simulink model "IEEE_1547_UI_TEST"  (R2018b)
settings: Solver=ode4  StartTime=0.0  StopTime=inf  FixedStep=Ts  RelTol=1e-3  EnableMultiTasking=on
PostLoadFcn:
  | Ts=40e-6; ARTEMIS_DISABLE_RTLAB_COMPATIBILTY_CHECK=1;
InitFcn:
  | Ts=40e-6; ARTEMIS_DISABLE_RTLAB_COMPATIBILTY_CHECK=1;
undefined symbols (not defined in the file or in its folder): another_event_name, I, Left, my_event_name, Right, type, V
libraries: simulink x72, powerlib_meascontrol x70, powerlib x66, artemis x4, rtlab x3, rtio_opalrt_ml605ex1 x3
(part 1 of 3)
Description:
  | Model of a simple control system for use iin training.
settings Model: ARTEMISmethode_block_infos=$$__separator__$$IEEE_P1547_TEST_V22/ARTEMIS Guide$$__separator__$$  Creator=Paul Baracos  LastModifiedBy=DETLDAQ
settings DataIOCC: LimitDataPoints=on  SaveFormat=Array  SaveOutput=off  SaveTime=off  SignalLoggingName=sigsOut
settings OptimizationCC: BlockReduction=off  BooleanDataType=off  OptimizeBlockIOStorage=off  BufferReuse=off  GlobalBufferReuse=off  ExpressionFolding=off  LocalBlockOutputs=off  InitFltsAndDblsToZero=on  LifeSpan=inf  OptimizeDataStoreBuffers=off  BusAssignmentInplaceUpdate=off
settings DebuggingCC: SaveWithParameterizedLinksMsg=none  UnderspecifiedInitializationDetection=Classic  MergeDetectMultiDrivingBlocksExec=none  SignalResolutionControl=TryResolveAllWithWarning  MultiTaskDSMMsg=warning  MultiTaskCondExecSysMsg=none  FcnCallInpInsideContextMsg=warning  SFUnexpectedBacktrackingDiag=warning  SFNoUnconditionalDefaultTransitionDiag=warning  SFExecutionAtInitializationDiag=none
settings HardwareCC: ProdBitPerPointer=32  ProdBitPerSizeT=32  ProdBitPerPtrDiffT=32  ProdLargestAtomicFloat=None  ProdIntDivRoundTo=Undefined  ProdEndianess=Unspecified  ProdWordSize=32  ProdHWDeviceType=32-bit Generic  TargetBitPerPointer=64  TargetBitPerSizeT=64  TargetBitPerPtrDiffT=64  TargetLongLongMode=on  TargetIntDivRoundTo=Zero  TargetEndianess=LittleEndian  TargetWordSize=64  TargetHWDeviceType=MATLAB Host  ProdEqTarget=off
settings ModelReferenceCC: PropagateSignalLabelsOutOfModel=off
settings SFSimCC: SimUseLocalCustomCode=off
settings RTWCC: Description=Generic Real-Time Target  RTWUseLocalCustomCode=off
settings CodeAppCC: StateflowObjectComments=on
settings GRTTargetCC: TargetFcnLib=ansi_tfl_tmw.mat  TargetLangStandard=C89/C90 (ANSI)  GeneratePreprocessorConditionals=Disable all  CombineOutputUpdateFcns=off  GRTInterface=on
settings ConfigComp: CovMetricSettings=dw  CovHtmlReporting=on  CovSaveCumulativeToWorkspaceVar=on  CovSaveSingleToWorkspaceVar=on  CovExternalEMLEnable=off

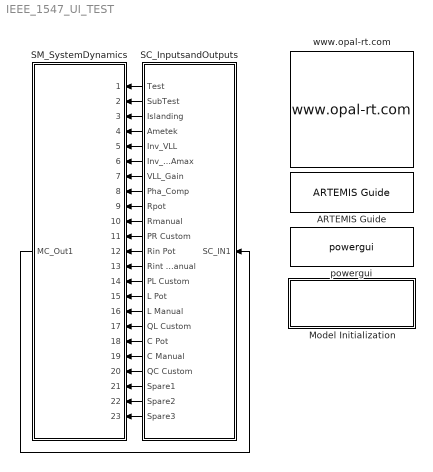
== system IEEE_1547_UI_TEST ==
  ARTEMIS Guide : artemis/ARTEMIS/ARTEMIS Guide  Tag=FTSSmethode_opal_4hx0r99  Description=5.0_z1  lock=on  Ts=Ts  ssn=on  opt=art5  dyna=off  nb_perm=4  RT_fullcomp=off  ssn_itvc=off  ssn_ivic=off  ssn_ext=off  ssn_solver=Backward Euler  iter_type=iSWITCH and iMOV only (default)  ssn_ImpulseLoopBlockedStateUpdate=5  ssn_mov_iter_number=5  ssn_switch_iter_number=5  ssn_lu_or_ldlt=LU (more robust)  ssn_nib_type_verify=on  ssn_use_lu=on  ssn_use_ldlt=off  ssn_impulse=on  ssn_quasimpulse=off  ssn_impulse_loop=5  paraExtinctionThy=off  Thy_Impulse=off  dtc=Off  dtc_opt=normal  ao=on  simtype=off  ct_mac=off  lin_mov=off  lsp=[0.001 2]  spike_skip=Disabled  dtc_extra=1  dtc_sws=normal  dtc_pied=0.5  SPSRulesBlock=SPSRules  tre=off  ctmm=off  LF=on  dpl_type=ARTEMiS DPL  rlc_type=off  custom_type=off  para=on  ssn_full_iteration=off
  Model Initialization : Subsystem  AncestorBlock=artemis/Tools /Misc/Model Initialization  mask(Model Functions){InitFcnX=Ts=40e-6; ARTEMIS_DISABLE_RTLAB_COMPATIBILTY_CHECK=1;, prel=off, posl=on, inif=on, strf=off}
      mask prompts: InitFcnX "Initialisation"; prel "Preload Function"; posl "PostLoad Function"; inif "InitFcn"; strf "StartFcn"
      mask init:
      | currentBlock = gcb;
      | root = bdroot(currentBlock);
      | 
      | if ~strcmp(get_param(root,'BlockDiagramType'),'library')
      |     if prel==1
      |         set_param(root, 'PreLoadFcn', InitFcnX);
      |     else
      |         set_param(root, 'PreLoadFcn', '');
      |     end
      |     if inif==1
      |         set_param(root, 'InitFcn', InitFcnX);
      |     else
      |         set_param(root, 'InitFcn', '');
      |     end
      |     if strf==1
      |         set_param(root, 'StartFcn', InitFcnX);
      |     else
      |         set_param(root, 'StartFcn', '');
      |     end
      |     if posl==1
      |         set_param(root, 'PostLoadFcn', InitFcnX);
      |     else
      |         set_param(root, 'PostLoadFcn', '');
      |     end
      | end
      | 
      | pos = get_param(currentBlock, 'Position');
      | width = pos(3) - pos(1); height = pos(4) - pos(2);
      | txt = [ upper(root) '\n' '- InitFcn. . . . . '  get_param(root, 'InitFcn') ];
      settings: CopyFcn=set_param(gcb,'LinkStatus','inactive')
      mask Display: text(5, height*0.5, txt, 'horizontalAlignment', 'left', 'verticalAlignment', 'middle') ;
  SC_InputsandOutputs : Subsystem
  SM_SystemDynamics : Subsystem
  powergui : powerlib/powergui  Priority=1  SimulationMode=Discrete  SampleTime=Ts  frequency=60  Iterations=50  frequencyindice=60  Pbase=100e6  ErrMax=1e-4  UnitsV=kV  UnitsW=MW  buscounter=0  FunctionMessages=off  echomessages=off  EnableUseOfTLC=off  CurrentSourceSwitches=off  DisableSnubberDevices=off  DisableRonSwitches=off  DisableVfSwitches=off  DisplayEquations=off  SolverType=Tustin/Backward Euler (TBE)  Interpol=off  ExternalGateDelay=off  methode=off  Ts=10  x0status=blocks  SPID=off  SwTol=0  HookPort=off  RestoreLinks=warning  ResistiveCurrentMeasurement=off  Frange=[0:2:500]  Ylog=off  Xlog=on  ShowGrid=off  save=off  variable=ZData  structure=0  ZoomFFT=off  StartTime=0.0  cycles=1  DisplayStyle=1  fundamental=60  FreqAxis=off  MaxFrequency=1000  frequencyindicesteady=1  RmsSteady=1  display=off
  www.opal-rt.com : artemis/Internal/www.opal-rt.com  SystemSampleTime=-1
  wires:
  SM_SystemDynamics/1(MC_Out1) -> SC_InputsandOutputs/1(SC_IN1)
  SC_InputsandOutputs/1(Test) -> SM_SystemDynamics/1(" 1")
  SC_InputsandOutputs/2(SubTest) -> SM_SystemDynamics/2(" 2")
  SC_InputsandOutputs/3(Islanding) -> SM_SystemDynamics/3(" 3")
  SC_InputsandOutputs/4(Ametek) -> SM_SystemDynamics/4(" 4")
  SC_InputsandOutputs/5(Inv_VLL) -> SM_SystemDynamics/5(" 5")
  SC_InputsandOutputs/6(Inv_KVAmax) -> SM_SystemDynamics/6(" 6")
  SC_InputsandOutputs/7(VLL_Gain) -> SM_SystemDynamics/7(" 7")
  SC_InputsandOutputs/8(Pha_Comp) -> SM_SystemDynamics/8(" 8")
  SC_InputsandOutputs/9(Rpot) -> SM_SystemDynamics/9(" 9")
  SC_InputsandOutputs/10(Rmanual) -> SM_SystemDynamics/10(" 10")
  SC_InputsandOutputs/11(PR Custom) -> SM_SystemDynamics/11(" 11")
  SC_InputsandOutputs/12(Rin Pot) -> SM_SystemDynamics/12(" 12")
  SC_InputsandOutputs/13(Rint Manual) -> SM_SystemDynamics/13(" 13")
  SC_InputsandOutputs/14(PL Custom) -> SM_SystemDynamics/14(" 14")
  SC_InputsandOutputs/15(L Pot) -> SM_SystemDynamics/15(" 15")
  SC_InputsandOutputs/16(L Manual) -> SM_SystemDynamics/16(" 16")
  SC_InputsandOutputs/17(QL Custom) -> SM_SystemDynamics/17(" 17")
  SC_InputsandOutputs/18(C Pot) -> SM_SystemDynamics/18(" 18")
  SC_InputsandOutputs/19(C Manual) -> SM_SystemDynamics/19(" 19")
  SC_InputsandOutputs/20(QC Custom) -> SM_SystemDynamics/20(" 20")
  SC_InputsandOutputs/21(Spare1) -> SM_SystemDynamics/21(" 21")
  SC_InputsandOutputs/22(Spare2) -> SM_SystemDynamics/22(" 22")
  SC_InputsandOutputs/23(Spare3) -> SM_SystemDynamics/23(" 23")

== system IEEE_1547_UI_TEST/Model Initialization ==

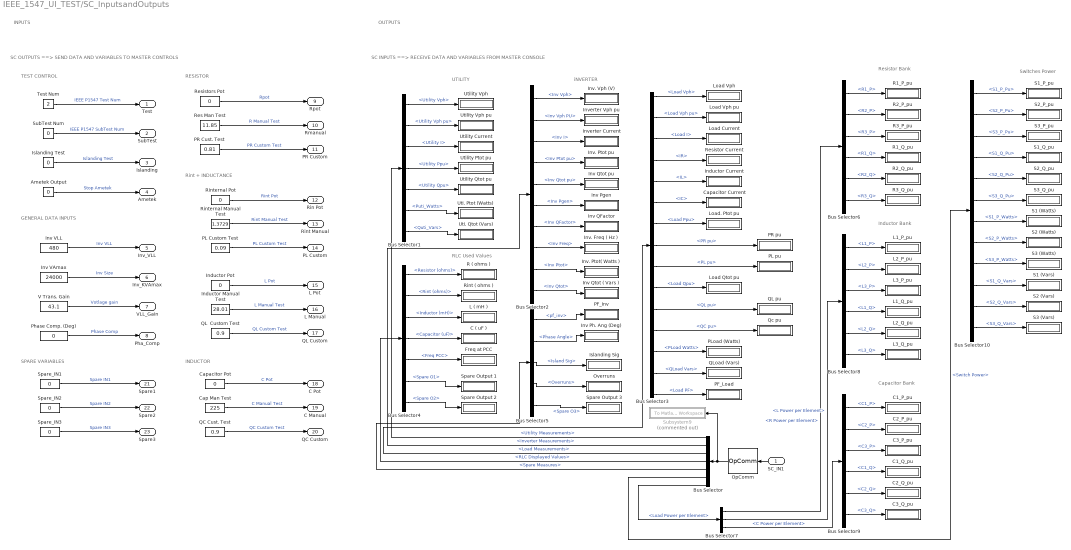
== system IEEE_1547_UI_TEST/SC_InputsandOutputs ==
  note: INPUTS
  note: RLC Used Values
  note: iNVERTER
  note: UTILITY
  note: SC INPUTS ==> RECEIVE DATA AND VARIABLES FROM MASTER CONSOLE
  note: TEST CONTROL
  note: SC OUTPUTS ==> SEND DATA AND VARIABLES TO MASTER CONTROLS
  note: INDUCTOR
  note: RESISTOR
  note: GENERAL DATA INPUTS
  note: Rint + INDUCTANCE
  note: SPARE VARIABLES
  note: OUTPUTS
  note: Resistor Bank
  note: Inductor Bank
  note: Capacitor Bank
  note: Switches Power
  SC_IN1 : Inport
  " PF_Load" : Display
  Ametek Output : Constant  Value=0
  Bus Selector : BusSelector  OutputSignals=Utility Measurements,Inverter Measurements,Load Measurements,RLC Displayed Values,Spare Measures,Switch Power,Load Power per Element
  Bus Selector1 : BusSelector  OutputSignals=Utility Vph,Utility Vph pu,Utility I,Utility Ppu,Utility Qpu,Puti_Watts,Quti_Vars
  Bus Selector10 : BusSelector  OutputSignals=S1_P_Pu,S2_P_Pu,S3_P_Pu,S1_Q_Pu,S2_Q_Pu,S3_Q_Pu,S1_P_Watts,S2_P_Watts,S3_P_Watts,S1_Q_Vars,S2_Q_Vars,S3_Q_Vars
  Bus Selector2 : BusSelector  OutputSignals=Inv Vph,Inv Vph PU,Inv I,Inv Ptot pu,Inv Qtot pu,Inv Pgen,Inv QFactor,Inv Freq,Inv Ptot,Inv Qtot
  Bus Selector3 : BusSelector  OutputSignals=Load Vph,Load Vph pu,Load I,IR,IL,IC,Load Ppu,PR pu,PL pu,Load Qpu,QL pu,QC pu,PLoad Watts,QLoad Vars,Load PF
  Bus Selector4 : BusSelector  OutputSignals=Resistor (ohms),Rint (ohms),Inductor (mH),Capacitor (uF),Freq PCC,Spare O1,Spare O2
  Bus Selector5 : BusSelector  OutputSignals=pf_inv,Phase Angle,Island Sig,Overruns,Spare O3
  Bus Selector6 : BusSelector  OutputSignals=R1_P,R2_P,R3_P,R1_Q,R2_Q,R3_Q
  Bus Selector7 : BusSelector  OutputSignals=R Power per Element,L Power per Element,C Power per Element
  Bus Selector8 : BusSelector  OutputSignals=L1_P,L2_P,L3_P,L1_Q,L2_Q,L3_Q
  Bus Selector9 : BusSelector  OutputSignals=C1_P,C2_P,C3_P,C1_Q,C2_Q,C3_Q
  C ( uF ) : Display
  C1_P_pu : Display
      settings: Format=bank
  C1_Q_pu : Display
  C2_P_pu : Display
  C2_Q_pu : Display
  C3_P_pu : Display
      settings: Format=bank
  C3_Q_pu : Display
      settings: Format=bank
  Cap Man Test : Constant  Value=225
  Capacitor Current : Display
      settings: Format=bank
  Capacitor Pot : Constant  Value=0
  Freq at PCC : Display
      settings: Format=bank
  Inductor Current : Display
      settings: Format=bank
  Inductor Manual Test : Constant  Value=28.01
  Inductor Pot : Constant  Value=0
  Inv Pgen : Display
  Inv Ph. Ang (Deg) : Display
  Inv QFactor : Display
  Inv Qtot ( Vars ) : Display
      settings: Format=bank
  Inv Qtot pu : Display
  Inv VAmax : Constant  Value=24000
  Inv VLL : Constant  Value=480
  Inv. Freq ( Hz ) : Display
      settings: Format=bank
  Inv. Ptot pu : Display
  Inv. Ptot( Watts ) : Display
      settings: Format=bank
  Inv. Vph (V) : Display
      settings: Format=bank
  Inverter Current : Display
      settings: Format=bank
  Inverter Vph pu : Display
  Islanding Sig : Display
  Islanding Test : Constant  Value=0
  L ( mH ) : Display
  L1_P_pu : Display
      settings: Format=bank
  L1_Q_pu : Display
  L2_P_pu : Display
  L2_Q_pu : Display
  L3_P_pu : Display
      settings: Format=bank
  L3_Q_pu : Display
      settings: Format=bank
  Load Current : Display
      settings: Format=bank
  Load Qtot pu : Display
  Load Vph : Display
      settings: Format=bank
  Load Vph pu : Display
  Load. Ptot pu : Display
  OpComm : rtlab/OpComm  nbport=1  groupe_acq=1  subsys_rate=0  st=0  Synchronization=on  Interpolation=on  Threshold=1.0  Missed_Data=off  Sim_Time=off  Samples=off  dynSigOut=off  from_console=0  warning_done=off  writeOpCommFile=off  Offset=off
      settings: SourceProductName=RT-LAB
  Overruns : Display
  PF_Inv : Display
  PL Custom Test : Constant  Value=0.09
  PL pu : Display
  PLoad (Watts) : Display
      settings: Format=bank
  PR Cust. Test : Constant  Value=0.81
  PR pu : Display
  Phase Comp. (Deg) : Constant  Value=0
  QC Cust. Test : Constant  Value=0.9
  QL  Custom Test : Constant  Value=0.9
  QL pu : Display
  QLoad (Vars) : Display
      settings: Format=bank
  Qc pu : Display
  R ( ohms ) : Display
  R1_P_pu : Display
      settings: Format=bank
  R1_Q_pu : Display
  R2_P_pu : Display
  R2_Q_pu : Display
  R3_P_pu : Display
      settings: Format=bank
  R3_Q_pu : Display
      settings: Format=bank
  Res Man Test : Constant  Value=11.85
  Resistor Current : Display
      settings: Format=bank
  Resistors Pot : Constant  Value=0
  Rint ( ohms ) : Display
  Rinternal Manual Test : Constant  Value=1.3729
  Rinternal Pot : Constant  Value=0
  S1 (Vars) : Display
  S1 (Watts) : Display
      settings: Format=bank
  S1_P_pu : Display
      settings: Format=bank
  S1_Q_pu : Display
  S2 (Vars) : Display
  S2 (Watts) : Display
      settings: Format=bank
  S2_P_pu : Display
      settings: Format=bank
  S2_Q_pu : Display
  S3 (Vars) : Display
      settings: Format=bank
  S3 (Watts) : Display
  S3_P_pu : Display
  S3_Q_pu : Display
      settings: Format=bank
  Spare Output 1 : Display
  Spare Output 2 : Display
  Spare Output 3 : Display
  Spare_IN1 : Constant  Value=0
  Spare_IN2 : Constant  Value=0
  Spare_IN3 : Constant  Value=0
  SubTest Num : Constant  Value=0
  Subsystem9 : Subsystem  Commented=on
  Test Num : Constant  Value=2
  Uti. Ptot (Watts) : Display
      settings: Format=bank
  Uti. Qtot (Vars) : Display
      settings: Format=bank
  Utility Current : Display
      settings: Format=bank
  Utility Ptot pu : Display
  Utility Qtot pu : Display
  Utility Vph : Display
      settings: Format=bank
  Utility Vph pu : Display
  V Trans. Gain : Constant  Value=43.1
  Test : Outport
  SubTest : Outport  Port=2
  Islanding : Outport  Port=3
  Ametek : Outport  Port=4
  Inv_VLL : Outport  Port=5
  Inv_KVAmax : Outport  Port=6
  VLL_Gain : Outport  Port=7
  Pha_Comp : Outport  Port=8
  Rpot : Outport  Port=9
  Rmanual : Outport  Port=10
  PR Custom : Outport  Port=11
  Rin Pot : Outport  Port=12
  Rint Manual : Outport  Port=13
  PL Custom : Outport  Port=14
  L Pot : Outport  Port=15
  L Manual : Outport  Port=16
  QL Custom : Outport  Port=17
  C Pot : Outport  Port=18
  C Manual : Outport  Port=19
  QC Custom : Outport  Port=20
  Spare1 : Outport  Port=21
  Spare2 : Outport  Port=22
  Spare3 : Outport  Port=23
  wires:
  SC_IN1/1 -> OpComm/1
  Bus Selector/1 -> Bus Selector1/1  "<Utility Measurements>"
  Bus Selector/2 -> Bus Selector2/1  "<Inverter Measurements>"
  Bus Selector/3 -> Bus Selector3/1  "<Load Measurements>"
  Bus Selector/4 -> Bus Selector4/1  "<RLC Displayed Values>"
  Bus Selector/5 -> Bus Selector5/1  "<Spare Measures>"
  Capacitor Pot/1 -> C Pot/1  "C Pot"
  QL  Custom Test/1 -> QL Custom/1  "QL Custom Test"
  Inductor Pot/1 -> L Pot/1  "L Pot"
  Res Man Test/1 -> Rmanual/1  "R Manual Test"
  PR Cust. Test/1 -> PR Custom/1  "PR Custom Test"
  Inductor Manual Test/1 -> L Manual/1  "L Manual Test"
  Rinternal Pot/1 -> Rin Pot/1  "Rint Pot"
  PL Custom Test/1 -> PL Custom/1  "PL Custom Test"
  Resistors Pot/1 -> Rpot/1  "Rpot"
  Rinternal Manual Test/1 -> Rint Manual/1  "Rint Manual Test"
  QC Cust. Test/1 -> QC Custom/1  "QC Custom Test"
  Cap Man Test/1 -> C Manual/1  "C Manual Test"
  Test Num/1 -> Test/1  "IEEE P1547 Test Num"
  SubTest Num/1 -> SubTest/1  "IEEE P1547 SubTest Num"
  Ametek Output/1 -> Ametek/1  "Stop Ametek"
  Islanding Test/1 -> Islanding/1  "Islanding Test"
  V Trans. Gain/1 -> VLL_Gain/1  "Votlage gain"
  Phase Comp. (Deg)/1 -> Pha_Comp/1  "Phase Comp"
  Inv VLL/1 -> Inv_VLL/1  "Inv VLL"
  Inv VAmax/1 -> Inv_KVAmax/1  "Inv Size"
  Spare_IN3/1 -> Spare3/1  "Spare IN3"
  Spare_IN1/1 -> Spare1/1  "Spare IN1"
  Spare_IN2/1 -> Spare2/1  "Spare IN2"
  Bus Selector1/2 -> Utility Vph pu/1  "<Utility Vph pu>"
  Bus Selector1/7 -> Uti. Qtot (Vars)/1  "<Quti_Vars>"
  Bus Selector1/6 -> Uti. Ptot (Watts)/1  "<Puti_Watts>"
  Bus Selector1/4 -> Utility Ptot pu/1  "<Utility Ppu>"
  Bus Selector1/3 -> Utility Current/1  "<Utility I>"
  Bus Selector1/5 -> Utility Qtot pu/1  "<Utility Qpu>"
  Bus Selector1/1 -> Utility Vph/1  "<Utility Vph>"
  Bus Selector2/6 -> Inv Pgen/1  "<Inv Pgen>"
  Bus Selector2/2 -> Inverter Vph pu/1  "<Inv Vph PU>"
  Bus Selector2/3 -> Inverter Current/1  "<Inv I>"
  Bus Selector2/9 -> Inv. Ptot( Watts )/1  "<Inv Ptot>"
  Bus Selector2/7 -> Inv QFactor/1  "<Inv QFactor>"
  Bus Selector2/10 -> Inv Qtot ( Vars )/1  "<Inv Qtot>"
  Bus Selector2/8 -> Inv. Freq ( Hz )/1  "<Inv Freq>"
  Bus Selector2/1 -> Inv. Vph (V)/1  "<Inv Vph>"
  Bus Selector2/4 -> Inv. Ptot pu/1  "<Inv Ptot pu>"
  Bus Selector2/5 -> Inv Qtot pu/1  "<Inv Qtot pu>"
  Bus Selector3/6 -> Capacitor Current/1  "<IC>"
  Bus Selector3/4 -> Resistor Current/1  "<IR>"
  Bus Selector3/7 -> Load. Ptot pu/1  "<Load Ppu>"
  Bus Selector3/15 -> " PF_Load"/1  "<Load PF>"
  Bus Selector3/10 -> Load Qtot pu/1  "<Load Qpu>"
  Bus Selector3/2 -> Load Vph pu/1  "<Load Vph pu>"
  Bus Selector3/3 -> Load Current/1  "<Load I>"
  Bus Selector3/9 -> PL pu/1  "<PL pu>"
  Bus Selector3/5 -> Inductor Current/1  "<IL>"
  Bus Selector3/11 -> QL pu/1  "<QL pu>"
  Bus Selector3/1 -> Load Vph/1  "<Load Vph>"
  Bus Selector3/12 -> Qc pu/1  "<QC pu>"
  Bus Selector3/8 -> PR pu/1  "<PR pu>"
  Bus Selector4/4 -> C ( uF )/1  "<Capacitor (uF)>"
  Bus Selector4/1 -> R ( ohms )/1  "<Resistor (ohms)>"
  Bus Selector4/3 -> L ( mH )/1  "<Inductor (mH)>"
  Bus Selector4/2 -> Rint ( ohms )/1  "<Rint (ohms)>"
  Bus Selector5/3 -> Islanding Sig/1  "<Island Sig>"
  Bus Selector5/5 -> Spare Output 3/1  "<Spare O3>"
  Bus Selector5/2 -> Inv Ph. Ang (Deg)/1  "<Phase Angle>"
  Bus Selector5/1 -> PF_Inv/1  "<pf_inv>"
  OpComm/1 -> Subsystem9/1(" To Matlab Workspace"), Bus Selector/1
  Bus Selector5/4 -> Overruns/1  "<Overruns>"
  Bus Selector4/5 -> Freq at PCC/1  "<Freq PCC>"
  Bus Selector4/6 -> Spare Output 1/1  "<Spare O1>"
  Bus Selector4/7 -> Spare Output 2/1  "<Spare O2>"
  Bus Selector3/13 -> PLoad (Watts)/1  "<PLoad Watts>"
  Bus Selector3/14 -> QLoad (Vars)/1  "<QLoad Vars>"
  Bus Selector7/1 -> Bus Selector6/1  "<R Power per Element>"
  Bus Selector6/6 -> R3_Q_pu/1  "<R3_Q>"
  Bus Selector8/6 -> L3_Q_pu/1  "<L3_Q>"
  Bus Selector/6 -> Bus Selector10/1  "<Switch Power>"
  Bus Selector6/1 -> R1_P_pu/1  "<R1_P>"
  Bus Selector8/4 -> L1_Q_pu/1  "<L1_Q>"
  Bus Selector7/3 -> Bus Selector9/1  "<C Power per Element>"
  Bus Selector7/2 -> Bus Selector8/1  "<L Power per Element>"
  Bus Selector8/1 -> L1_P_pu/1  "<L1_P>"
  Bus Selector9/4 -> C1_Q_pu/1  "<C1_Q>"
  Bus Selector9/5 -> C2_Q_pu/1  "<C2_Q>"
  Bus Selector9/1 -> C1_P_pu/1  "<C1_P>"
  Bus Selector6/2 -> R2_P_pu/1  "<R2_P>"
  Bus Selector6/3 -> R3_P_pu/1  "<R3_P>"
  Bus Selector6/4 -> R1_Q_pu/1  "<R1_Q>"
  Bus Selector8/5 -> L2_Q_pu/1  "<L2_Q>"
  Bus Selector9/2 -> C2_P_pu/1  "<C2_P>"
  Bus Selector8/3 -> L3_P_pu/1  "<L3_P>"
  Bus Selector8/2 -> L2_P_pu/1  "<L2_P>"
  Bus Selector9/6 -> C3_Q_pu/1  "<C3_Q>"
  Bus Selector9/3 -> C3_P_pu/1  "<C3_P>"
  Bus Selector6/5 -> R2_Q_pu/1  "<R2_Q>"
  Bus Selector/7 -> Bus Selector7/1  "<Load Power per Element>"
  Bus Selector10/5 -> S2_Q_pu/1  "<S2_Q_Pu>"
  Bus Selector10/2 -> S2_P_pu/1  "<S2_P_Pu>"
  Bus Selector10/11 -> S2 (Vars)/1  "<S2_Q_Vars>"
  Bus Selector10/4 -> S1_Q_pu/1  "<S1_Q_Pu>"
  Bus Selector10/8 -> S2 (Watts)/1  "<S2_P_Watts>"
  Bus Selector10/3 -> S3_P_pu/1  "<S3_P_Pu>"
  Bus Selector10/9 -> S3 (Watts)/1  "<S3_P_Watts>"
  Bus Selector10/10 -> S1 (Vars)/1  "<S1_Q_Vars>"
  Bus Selector10/1 -> S1_P_pu/1  "<S1_P_Pu>"
  Bus Selector10/12 -> S3 (Vars)/1  "<S3_Q_Vars>"
  Bus Selector10/6 -> S3_Q_pu/1  "<S3_Q_Pu>"
  Bus Selector10/7 -> S1 (Watts)/1  "<S1_P_Watts>"

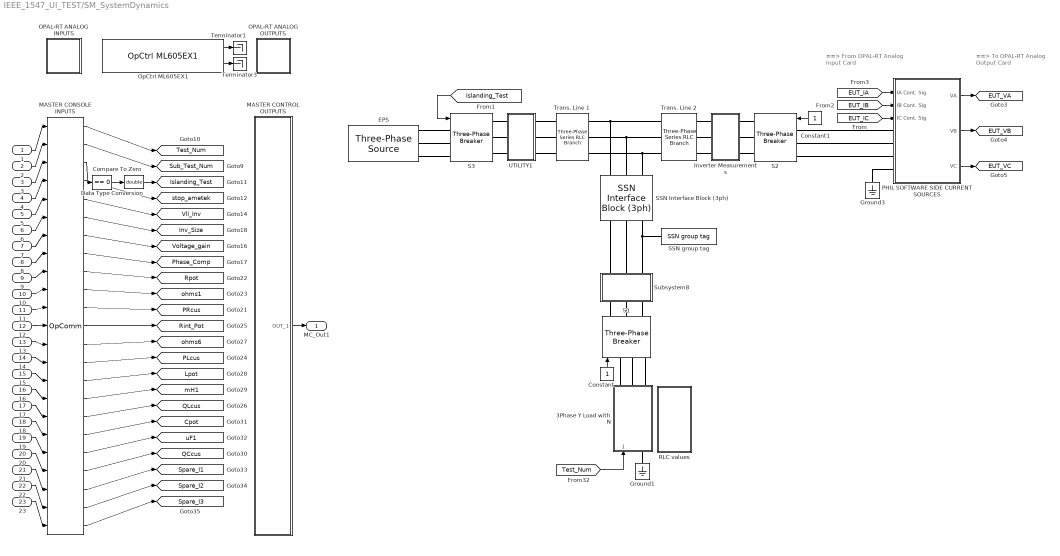
== system IEEE_1547_UI_TEST/SM_SystemDynamics ==
  note: ==> From OPAL-RT
      | Analog Input
      | Card
  note: ==> To OPAL-RT
      | Analog Output
      | Card
  " 1" : Inport
  " 2" : Inport  Port=2
  " 3" : Inport  Port=3
  " 4" : Inport  Port=4
  " 5" : Inport  Port=5
  " 6" : Inport  Port=6
  " 7" : Inport  Port=7
  " 8" : Inport  Port=8
  " 9" : Inport  Port=9
  " 10" : Inport  Port=10
  " 11" : Inport  Port=11
  " 12" : Inport  Port=12
  " 13" : Inport  Port=13
  " 14" : Inport  Port=14
  " 15" : Inport  Port=15
  " 16" : Inport  Port=16
  " 17" : Inport  Port=17
  " 18" : Inport  Port=18
  " 19" : Inport  Port=19
  " 20" : Inport  Port=20
  " 21" : Inport  Port=21
  " 22" : Inport  Port=22
  " 23" : Inport  Port=23
  " 3Phase Y Load with N" : Subsystem
      mask Display:
      | color('blue');
      | disp('3Phase\nY Load\nwith N\n\n');
  " EPS " : powerlib/Electrical Sources/Three-Phase Source  InternalConnection=Yg  VoltagePhases=off  Voltage=480  PhaseAngle=0  Voltage_phases=[613 613 613]/sqrt(3)  PhaseAngles_phases=[30 -90 +150]  Frequency=60  NonIdealSource=on  SpecifyImpedance=on  Resistance=0.002957  Inductance=0.000031  ShortCircuitLevel=1e6  BaseVoltage=480  XRratio=7  BusType=swing  Pref=10e3  Qref=0  Prefabc=[10e3, 10e3, 10e3]  Qrefabc=[0, 0, 0]  Qmin=-inf  Qmax=inf
      settings: SourceProductName=Simscape Electrical
  Compare To Zero : simulink/Logic and Bit Operations/Compare To Zero  relop===  OutDataTypeStr=boolean
  Constant : Constant
  Constant1 : Constant
  Data Type Conversion : DataTypeConversion  OutDataTypeStr=double
  Ground1 : powerlib/Elements/Ground  LConnTagsString=a
      settings: SourceProductName=Simscape Electrical
  Ground3 : powerlib/Elements/Ground  LConnTagsString=a
      settings: SourceProductName=Simscape Electrical
  Inverter Measurements : Subsystem
      mask Display:
      | % color('blue')
      | % disp('Inverter\nMeasurements')
  MASTER CONSOLE INPUTS : rtlab/OpComm  nbport=23  groupe_acq=1  subsys_rate=0  st=0  Synchronization=on  Interpolation=on  Threshold=1.0  Missed_Data=off  Sim_Time=off  Samples=off  dynSigOut=off  from_console=1  warning_done=off  writeOpCommFile=off  Offset=off
      settings: SourceProductName=RT-LAB
  MASTER CONTROL OUTPUTS : Subsystem
  OPAL-RT ANALOG INPUTS : Subsystem
      mask Display:
      | color('red')
      | disp('\nOpal-RT\n\n\n')
      | color('blue')
      | disp('\nAI\nCard')
  OPAL-RT ANALOG OUTPUTS : Subsystem
      mask Display:
      | color('red')
      | disp('\nOpal-RT\n\n\n')
      | color('blue')
      | disp('\nAO\nCard')
  OpCtrl ML605EX1 : rtio_opalrt_ml605ex1/OpCtrl ML605EX1  CtrlName='ML605EX1 Ctrl'  boardid=0  BitstreamFilename=ML605_2-EX-0029-2_3_7_140-32Ao_16Ai_32DioSelectable_C3C1C3FBFBEA-01-05.bin  numconfig=-1  mode=Master  externalClock=off  decimRtsi=0  calibIO=off  SampleTime=0  loadinport=-1
  PHIL SOFTWARE SIDE CURRENT SOURCES : Subsystem
      mask Display:
      | color('blue')
      | disp('\nPHIL\nInverter')
      | color('red')
      | disp('\n\n\n\n\n\nY Grounded\nNeutral')
  RLC values : Subsystem
      mask Display:
      | color('blue')
      | disp('RLC\nValues')
  S1 : powerlib/Elements/Three-Phase Breaker  InitialState=closed  SwitchA=on  SwitchB=on  SwitchC=on  SwitchTimes="[1/60  5/60]"  External=on  BreakerResistance=0.01  SnubberResistance=1e6  SnubberCapacitance=inf  Measurements=None
      settings: SourceProductName=Simscape Electrical
  S2 : powerlib/Elements/Three-Phase Breaker  InitialState=closed  SwitchA=on  SwitchB=on  SwitchC=on  SwitchTimes="[1/60  5/60]"  External=on  BreakerResistance=0.01  SnubberResistance=1e6  SnubberCapacitance=inf  Measurements=None
      settings: SourceProductName=Simscape Electrical
  "S3 " : powerlib/Elements/Three-Phase Breaker  InitialState=closed  SwitchA=on  SwitchB=on  SwitchC=on  SwitchTimes="[1/60  5/60]"  External=on  BreakerResistance=0.01  SnubberResistance=1e6  SnubberCapacitance=inf  Measurements=None
      settings: SourceProductName=Simscape Electrical
  SSN Interface Block (3ph) : artemis/SSN/Nodal Interface Blocks/SSN Interface Block (3ph)  nb_phase=3  nb_port=2  p1_type=V-type(Left)  p2_type=I-type(Right)  p3_type=V-type(Left)  p4_type=V-type(Left)  p5_type=V-type(Left)  p6_type=V-type(Left)  p7_type=V-type(Left)  p8_type=V-type(Left)  p9_type=V-type(Left)  p10_type=V-type(Left)  p11_type=V-type(Left)  p12_type=V-type(Left)  p13_type=V-type(Left)  p14_type=V-type(Left)  p15_type=V-type(Left)  p16_type=V-type(Left)  I_port_shunt_resistance=1e9
  SSN group tag : artemis/SSN/SSN group tag  ssn_group_tag=Group2
  Subsystem8 : Subsystem
  Terminator1 : Terminator
  Terminator3 : Terminator
  Trans. Line 1 : powerlib/Elements/Three-Phase Series RLC Branch  LConnTagsString=A|B|C  RConnTagsString=A|B|C  BranchType=R  Resistance=0.014875  Inductance=0.0000855  Capacitance=1e-6  Measurements=None
      settings: SourceProductName=Simscape Electrical
  Trans. Line 2 : powerlib/Elements/Three-Phase Series RLC Branch  LConnTagsString=A|B|C  RConnTagsString=A|B|C  BranchType=R  Resistance=0.014875  Inductance=0.0000855  Capacitance=0  Measurements=None
      settings: SourceProductName=Simscape Electrical
  UTILITY1 : Subsystem
      mask Display:
      | % color('blue')
      | % disp('Utility\n\n')
      | % color('red')
      | % disp('\nY Grounded\nNeutral')
  MC_Out1 : Outport
  tag scope: Cpot=global, EUT_VA=global, EUT_VB=global, EUT_VC=global, Inv_Size=global, Islanding_Test=global, Lpot=global, PLcus=global, PRcus=global, Phase_Comp=global, QCcus=global, QLcus=global, Rint_Pot=global, Rpot=global, Spare_I1=global, Spare_I2=global, Spare_I3=global, Sub_Test_Num=global, Test_Num=global, Vll_Inv=global, Voltage_gain=global, mH1=global, ohms1=global, ohms6=global, stop_ametek=global, uF1=global
  wires:
  [Islanding_Test] -> "S3 "/1
  OpCtrl ML605EX1/1 -> Terminator1/1
  OpCtrl ML605EX1/2 -> Terminator3/1
  [EUT_IB] -> PHIL SOFTWARE SIDE CURRENT SOURCES/2(IB Cont. Sig)
  PHIL SOFTWARE SIDE CURRENT SOURCES/1(VA) -> [EUT_VA]
  PHIL SOFTWARE SIDE CURRENT SOURCES/2(VB) -> [EUT_VB]
  PHIL SOFTWARE SIDE CURRENT SOURCES/3(VC) -> [EUT_VC]
  [EUT_IA] -> PHIL SOFTWARE SIDE CURRENT SOURCES/1(IA Cont. Sig)
  [EUT_IC] -> PHIL SOFTWARE SIDE CURRENT SOURCES/3(IC Cont. Sig)
  [Test_Num] -> " 3Phase Y Load with N"/1(Test Sel.)
  " 1"/1 -> MASTER CONSOLE INPUTS/1
  " 4"/1 -> MASTER CONSOLE INPUTS/4
  " 2"/1 -> MASTER CONSOLE INPUTS/2
  " 3"/1 -> MASTER CONSOLE INPUTS/3
  " 5"/1 -> MASTER CONSOLE INPUTS/5
  " 6"/1 -> MASTER CONSOLE INPUTS/6
  " 7"/1 -> MASTER CONSOLE INPUTS/7
  " 8"/1 -> MASTER CONSOLE INPUTS/8
  " 9"/1 -> MASTER CONSOLE INPUTS/9
  " 10"/1 -> MASTER CONSOLE INPUTS/10
  " 11"/1 -> MASTER CONSOLE INPUTS/11
  " 12"/1 -> MASTER CONSOLE INPUTS/12
  " 13"/1 -> MASTER CONSOLE INPUTS/13
  " 14"/1 -> MASTER CONSOLE INPUTS/14
  " 15"/1 -> MASTER CONSOLE INPUTS/15
  " 16"/1 -> MASTER CONSOLE INPUTS/16
  " 17"/1 -> MASTER CONSOLE INPUTS/17
  " 18"/1 -> MASTER CONSOLE INPUTS/18
  " 19"/1 -> MASTER CONSOLE INPUTS/19
  " 20"/1 -> MASTER CONSOLE INPUTS/20
  " 21"/1 -> MASTER CONSOLE INPUTS/21
  " 22"/1 -> MASTER CONSOLE INPUTS/22
  " 23"/1 -> MASTER CONSOLE INPUTS/23
  MASTER CONSOLE INPUTS/1 -> [Test_Num]
  MASTER CONSOLE INPUTS/2 -> [Sub_Test_Num]
  MASTER CONSOLE INPUTS/4 -> [stop_ametek]
  MASTER CONSOLE INPUTS/5 -> [Vll_Inv]
  MASTER CONSOLE INPUTS/6 -> [Inv_Size]
  MASTER CONSOLE INPUTS/7 -> [Voltage_gain]
  MASTER CONSOLE INPUTS/8 -> [Phase_Comp]
  MASTER CONSOLE INPUTS/9 -> [Rpot]
  MASTER CONSOLE INPUTS/10 -> [ohms1]
  MASTER CONSOLE INPUTS/11 -> [PRcus]
  MASTER CONSOLE INPUTS/12 -> [Rint_Pot]
  MASTER CONSOLE INPUTS/13 -> [ohms6]
  MASTER CONSOLE INPUTS/14 -> [PLcus]
  MASTER CONSOLE INPUTS/15 -> [Lpot]
  MASTER CONSOLE INPUTS/16 -> [mH1]
  MASTER CONSOLE INPUTS/17 -> [QLcus]
  MASTER CONSOLE INPUTS/18 -> [Cpot]
  MASTER CONSOLE INPUTS/19 -> [uF1]
  MASTER CONSOLE INPUTS/20 -> [QCcus]
  MASTER CONSOLE INPUTS/21 -> [Spare_I1]
  MASTER CONSOLE INPUTS/22 -> [Spare_I2]
  MASTER CONSOLE INPUTS/23 -> [Spare_I3]
  MASTER CONTROL OUTPUTS/1("OUT_1 ") -> MC_Out1/1
  MASTER CONSOLE INPUTS/3 -> Compare To Zero/1
  Compare To Zero/1 -> Data Type Conversion/1
  Data Type Conversion/1 -> [Islanding_Test]
  Constant/1 -> S1/1
  Constant1/1 -> S2/1
  connections:
  Trans. Line 1/RConn1 -- Trans. Line 2/LConn1 -- SSN Interface Block (3ph)/LConn1
  Trans. Line 2/LConn2 -- Trans. Line 1/RConn2 -- SSN Interface Block (3ph)/LConn2
  Trans. Line 2/LConn3 -- Trans. Line 1/RConn3 -- SSN Interface Block (3ph)/LConn3
  Trans. Line 2/RConn1 -- Inverter Measurements/RConn1
  S2/RConn2 -- Inverter Measurements/LConn2
  Trans. Line 2/RConn2 -- Inverter Measurements/RConn2
  S2/RConn3 -- Inverter Measurements/LConn3
  Trans. Line 2/RConn3 -- Inverter Measurements/RConn3
  Ground3/LConn1 -- PHIL SOFTWARE SIDE CURRENT SOURCES/LConn4
  Subsystem8/LConn1 -- SSN Interface Block (3ph)/RConn1
  Subsystem8/LConn2 -- SSN Interface Block (3ph)/RConn2
  SSN group tag/LConn1 -- SSN Interface Block (3ph)/RConn3 -- Subsystem8/LConn3
  Ground1/LConn1 -- " 3Phase Y Load with N"/LConn1
  Subsystem8/RConn1 -- S1/RConn1
  Subsystem8/RConn2 -- S1/RConn2
  Subsystem8/RConn3 -- S1/RConn3
  S2/RConn1 -- Inverter Measurements/LConn1
  " 3Phase Y Load with N"/RConn1 -- S1/LConn1
  " 3Phase Y Load with N"/RConn2 -- S1/LConn2
  " 3Phase Y Load with N"/RConn3 -- S1/LConn3
  "S3 "/LConn1 -- " EPS "/RConn1
  "S3 "/LConn2 -- " EPS "/RConn2
  "S3 "/LConn3 -- " EPS "/RConn3
  UTILITY1/RConn1 -- Trans. Line 1/LConn1
  UTILITY1/RConn2 -- Trans. Line 1/LConn2
  UTILITY1/RConn3 -- Trans. Line 1/LConn3
  UTILITY1/LConn1 -- "S3 "/RConn1
  UTILITY1/LConn2 -- "S3 "/RConn2
  UTILITY1/LConn3 -- "S3 "/RConn3
  S2/LConn1 -- PHIL SOFTWARE SIDE CURRENT SOURCES/LConn1
  S2/LConn2 -- PHIL SOFTWARE SIDE CURRENT SOURCES/LConn2
  S2/LConn3 -- PHIL SOFTWARE SIDE CURRENT SOURCES/LConn3

== system IEEE_1547_UI_TEST/SC_InputsandOutputs/Subsystem9 ==
  " To Matlab Workspace" : Inport
  Bus Selector : BusSelector  OutputSignals=Utility Measurements,Inverter Measurements,Load Measurements,RLC Display Values
  Subsystem5 : Subsystem
  Subsystem6 : Subsystem
  Subsystem7 : Subsystem
  Subsystem8 : Subsystem
  wires:
  " To Matlab Workspace"/1 -> Bus Selector/1
  Bus Selector/2 -> Subsystem6/1(Inverter Measurements)  "<Inverter Measurements>"
  Bus Selector/1 -> Subsystem5/1(Utility Measurements)  "<Utility Measurements>"
  Bus Selector/3 -> Subsystem7/1(Load Measurements)  "<Load Measurements>"
  Bus Selector/4 -> Subsystem8/1(RLC Display Values)  "<RLC Display Values>"

== system IEEE_1547_UI_TEST/SM_SystemDynamics/ 3Phase Y Load with N ==
  Test Sel. : Inport
  "   C Bank" : Subsystem
  "   R Bank1" : Subsystem
  ( Rint + L ) Bank : Subsystem
  3Ph CB Normal : powerlib/Elements/Three-Phase Breaker  InitialState=closed  SwitchA=on  SwitchB=on  SwitchC=on  SwitchTimes="[1/60  5/60]"  External=on  BreakerResistance=0.01  SnubberResistance=1e6  SnubberCapacitance=inf  Measurements=None
      settings: SourceProductName=Simscape Electrical
  3Ph CB Test 1 : powerlib/Elements/Three-Phase Breaker  InitialState=closed  SwitchA=on  SwitchB=on  SwitchC=on  SwitchTimes="[1/60  5/60]"  External=on  BreakerResistance=0.01  SnubberResistance=1e6  SnubberCapacitance=inf  Measurements=None
      settings: SourceProductName=Simscape Electrical
  3Ph CB Test 2 : powerlib/Elements/Three-Phase Breaker  InitialState=closed  SwitchA=on  SwitchB=on  SwitchC=on  SwitchTimes="[1/60  5/60]"  External=on  BreakerResistance=0.01  SnubberResistance=1e6  SnubberCapacitance=inf  Measurements=None
      settings: SourceProductName=Simscape Electrical
  A : PMIOPort  Side=Right
  B : PMIOPort  Port=2  Side=Right
  C : PMIOPort  Port=3  Side=Right
  Ground : PMIOPort  Port=4  Side=Left
  tag scope: P_L=global, P_RL=global, Q_C=global, Q_L=global
  wires:
  [mH2] -> ( Rint + L ) Bank/1(mH)
  [ohms7] -> ( Rint + L ) Bank/2(Rint)
  ( Rint + L ) Bank/2(Q_L) -> [Q_L]
  [uF2] -> "   C Bank"/1(uC.)
  "   C Bank"/2(Q_C) -> [Q_C]
  ( Rint + L ) Bank/1(P_L) -> [P_L]
  "   R Bank1"/1(P_RL) -> [P_RL]
  [ohms2] -> "   R Bank1"/1(ohms)
  Test Sel./1 -> 3Ph CB Normal/1, 3Ph CB Test 2/1, 3Ph CB Test 1/1
  connections:
  B/RConn1 -- 3Ph CB Test 2/RConn2 -- 3Ph CB Test 1/RConn2 -- 3Ph CB Normal/RConn2
  C/RConn1 -- 3Ph CB Test 2/RConn3 -- 3Ph CB Test 1/RConn3 -- 3Ph CB Normal/RConn3
  3Ph CB Normal/LConn1 -- "   R Bank1"/LConn1
  3Ph CB Normal/LConn3 -- "   R Bank1"/LConn3
  3Ph CB Normal/LConn2 -- "   R Bank1"/LConn2
  3Ph CB Test 1/LConn2 -- ( Rint + L ) Bank/LConn2
  3Ph CB Test 1/LConn1 -- ( Rint + L ) Bank/LConn1
  3Ph CB Test 1/LConn3 -- ( Rint + L ) Bank/LConn3
  "   R Bank1"/RConn2 -- ( Rint + L ) Bank/RConn2 -- "   C Bank"/RConn2 -- "   C Bank"/RConn3 -- "   C Bank"/RConn1 -- "   R Bank1"/RConn3 -- ( Rint + L ) Bank/RConn3 -- Ground/RConn1 -- ( Rint + L ) Bank/RConn1 -- "   R Bank1"/RConn1
  A/RConn1 -- 3Ph CB Test 2/RConn1 -- 3Ph CB Test 1/RConn1 -- 3Ph CB Normal/RConn1
  3Ph CB Test 2/LConn1 -- "   C Bank"/LConn1
  3Ph CB Test 2/LConn2 -- "   C Bank"/LConn2
  3Ph CB Test 2/LConn3 -- "   C Bank"/LConn3

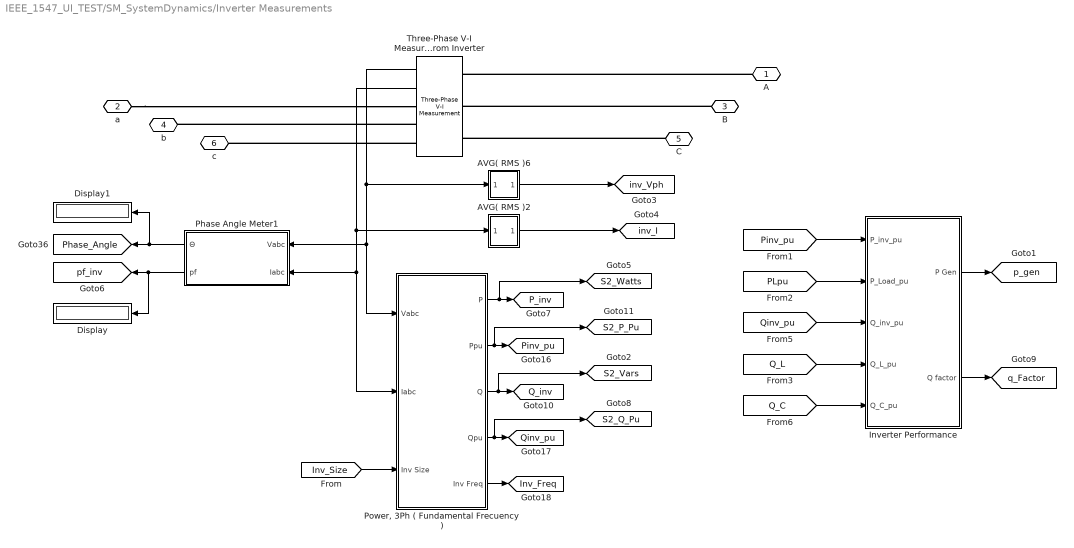
== system IEEE_1547_UI_TEST/SM_SystemDynamics/Inverter Measurements ==
  AVG( RMS )2 : Subsystem
      mask Display: color('blue');disp('RMS\nAVG')
  AVG( RMS )6 : Subsystem
      mask Display: color('blue');disp('RMS\nAVG')
  Display : Display
  Display1 : Display
  Inverter Performance : Subsystem
  Phase Angle Meter1 : Subsystem
      mask Display:
      | color('blue')
      | disp('Θ = (Θv - Θi)')
  "Power, 3Ph ( Fundamental Frecuency )" : Subsystem
  Three-Phase V-I Measurement From Inverter : powerlib/Measurements/Three-Phase V-I Measurement  VoltageMeasurement=phase-to-ground  SetLabelV=off  LabelV=Vabc_INV  Vpu=off  VpuLL=off  CurrentMeasurement=yes  SetLabelI=off  LabelI=Iabc_INV  Ipu=off  Pbase=100e6  Vbase=500e3  OutputType=Complex  PhasorSimulation=off  PSBequivalent=0
      settings: SourceProductName=Simscape Electrical
  A : PMIOPort  Side=Left
  a : PMIOPort  Port=2  Side=Right
  B : PMIOPort  Port=3  Side=Left
  b : PMIOPort  Port=4  Side=Right
  C : PMIOPort  Port=5  Side=Left
  c : PMIOPort  Port=6  Side=Right
  tag scope: Inv_Freq=global, P_inv=global, Phase_Angle=global, Pinv_pu=global, Q_inv=global, Qinv_pu=global, S2_P_Pu=global, S2_Q_Pu=global, S2_Vars=global, S2_Watts=global, inv_I=global, inv_Vph=global, p_gen=global, pf_inv=global, q_Factor=global
  wires:
  AVG( RMS )6/1(Out1) -> [inv_Vph]
  AVG( RMS )2/1(Out1) -> [inv_I]
  [Inv_Size] -> "Power, 3Ph ( Fundamental Frecuency )"/3(Inv Size)
  Three-Phase V-I Measurement From Inverter/1 -> AVG( RMS )6/1(In1), "Power, 3Ph ( Fundamental Frecuency )"/1(Vabc), Phase Angle Meter1/1(Vabc)
  Phase Angle Meter1/2(pf) -> Display/1, [pf_inv]
  Phase Angle Meter1/1(Θ) -> Display1/1, [Phase_Angle]
  Three-Phase V-I Measurement From Inverter/2 -> AVG( RMS )2/1(In1), "Power, 3Ph ( Fundamental Frecuency )"/2(Iabc), Phase Angle Meter1/2(Iabc)
  [Q_L] -> Inverter Performance/4(Q_L_pu)
  Inverter Performance/1(P Gen) -> [p_gen]
  Inverter Performance/2(Q factor) -> [q_Factor]
  [PLpu] -> Inverter Performance/2(P_Load_pu)
  [Pinv_pu] -> Inverter Performance/1(P_inv_pu)
  [Qinv_pu] -> Inverter Performance/3(Q_inv_pu)
  [Q_C] -> Inverter Performance/5(Q_C_pu)
  "Power, 3Ph ( Fundamental Frecuency )"/4(Qpu) -> [S2_Q_Pu], [Qinv_pu]
  "Power, 3Ph ( Fundamental Frecuency )"/3(Q) -> [S2_Vars], [Q_inv]
  "Power, 3Ph ( Fundamental Frecuency )"/2(Ppu) -> [S2_P_Pu], [Pinv_pu]
  "Power, 3Ph ( Fundamental Frecuency )"/1(P) -> [S2_Watts], [P_inv]
  "Power, 3Ph ( Fundamental Frecuency )"/5(Inv Freq) -> [Inv_Freq]
  connections:
  A/RConn1 -- Three-Phase V-I Measurement From Inverter/LConn1
  B/RConn1 -- Three-Phase V-I Measurement From Inverter/LConn2
  C/RConn1 -- Three-Phase V-I Measurement From Inverter/LConn3
  a/RConn1 -- Three-Phase V-I Measurement From Inverter/RConn1
  Three-Phase V-I Measurement From Inverter/RConn2 -- b/RConn1
  Three-Phase V-I Measurement From Inverter/RConn3 -- c/RConn1

== system IEEE_1547_UI_TEST/SM_SystemDynamics/MASTER CONTROL OUTPUTS ==
  Bus Creator : BusCreator  Inputs=7
  INVERTER MEASURES : Subsystem
  LOAD MEASURES : Subsystem
  RLC DISPLAYED VALUES : Subsystem
  SPARE MEASURES : Subsystem
  SPARE MEASURES1 : Subsystem
  SPARE MEASURES2 : Subsystem
  UTILITY MEASURES : Subsystem
  "OUT_1 " : Outport
  wires:
  RLC DISPLAYED VALUES/1(RLC Displayed Values) -> Bus Creator/6  "RLC Displayed Values"
  UTILITY MEASURES/1(Utility Measures) -> Bus Creator/1  "Utility Measurements"
  LOAD MEASURES/1(Load Measures) -> Bus Creator/3  "Load Measurements"
  INVERTER MEASURES/1(Inverter Measures) -> Bus Creator/2  "Inverter Measurements"
  SPARE MEASURES/1(Spare Measures) -> Bus Creator/7  "Spare Measures"
  Bus Creator/1 -> "OUT_1 "/1
  SPARE MEASURES1/1(Load Power per Element) -> Bus Creator/4  "Load Power per Element"
  SPARE MEASURES2/1(Switch Power) -> Bus Creator/5  "Switch Power"

== system IEEE_1547_UI_TEST/SM_SystemDynamics/OPAL-RT ANALOG INPUTS ==
  Demux : Demux  Outputs=8
  Inputs Signal Conditioning Circuit : Subsystem
  ML605EX1 AnalogIn : rtio_opalrt_ml605ex1/ML605EX1 AnalogIn  CtrlName='ML605EX1 Ctrl'  portNb=2  FcnNos=Slot 1 Module B Subsection 2  size=16  maxcount=8  count=8  numchan=8  sampleTime=0
      settings: AttributesFormatString=%<CtrlName>
  Terminator{2,4..7,9} (6 alike) : Terminator
  tag scope: EUT_IA=global, EUT_IB=global, EUT_IC=global
  wires:
  Demux/7 -> Inputs Signal Conditioning Circuit/5(I14 - VC in)
  Demux/6 -> Inputs Signal Conditioning Circuit/4(I13 - IB in)
  Inputs Signal Conditioning Circuit/5(" O14") -> Terminator7/1
  ML605EX1 AnalogIn/2 -> Terminator6/1
  ML605EX1 AnalogIn/1 -> Demux/1
  Inputs Signal Conditioning Circuit/2("O11 ") -> [EUT_IA]
  Demux/5 -> Inputs Signal Conditioning Circuit/3(I12 - VB in)
  Inputs Signal Conditioning Circuit/3(" O12") -> Terminator5/1
  Demux/4 -> Inputs Signal Conditioning Circuit/2(I11 - IA in)
  Demux/3 -> Inputs Signal Conditioning Circuit/1(I10 - VA in)
  Demux/2 -> Terminator2/1
  Demux/8 -> Inputs Signal Conditioning Circuit/6(I15 - IC in)
  Demux/1 -> Terminator9/1
  Inputs Signal Conditioning Circuit/4(" O13") -> [EUT_IB]
  Inputs Signal Conditioning Circuit/1("O10 ") -> Terminator4/1
  Inputs Signal Conditioning Circuit/6(" O15") -> [EUT_IC]

== system IEEE_1547_UI_TEST/SM_SystemDynamics/OPAL-RT ANALOG OUTPUTS ==
  Constant{,1..3} (4 alike) : Constant  Value=0
  ML605EX1 AnalogOut : rtio_opalrt_ml605ex1/ML605EX1 AnalogOut  CtrlName='ML605EX1 Ctrl'  portNb=1  FcnNos=Slot 1 Module A Subsection 1  size=16  maxcount=8  count=8  numchan=8  israngeinput=off  voltagerange=[-16 ... 16]  slot=0  side=0  mismatch=0  slotside=Slot_1_Module_A
      settings: AttributesFormatString=%<CtrlName>
  Mux1 : Mux  Inputs=8
  Outputs Signa Conditioning Circuit : Subsystem
  Terminator : Terminator
  wires:
  [Islanding_Test] -> Outputs Signa Conditioning Circuit/5(I4 - ISL. TRIGG.)
  Constant2/1 -> Outputs Signa Conditioning Circuit/7(I6 - N/C)
  Outputs Signa Conditioning Circuit/2(Out 1) -> Mux1/2
  ML605EX1 AnalogOut/1 -> Terminator/1
  Constant/1 -> Outputs Signa Conditioning Circuit/4(I3 - N/C)
  Outputs Signa Conditioning Circuit/7(Out 6) -> Mux1/7
  [EUT_VB] -> Outputs Signa Conditioning Circuit/2(I1 - VB)
  [EUT_VC] -> Outputs Signa Conditioning Circuit/3(I2 - VC)
  Mux1/1 -> ML605EX1 AnalogOut/1
  Outputs Signa Conditioning Circuit/3(Out 2) -> Mux1/3
  Outputs Signa Conditioning Circuit/5(Out 4) -> Mux1/5
  Outputs Signa Conditioning Circuit/4(Out 3) -> Mux1/4
  [EUT_VA] -> Outputs Signa Conditioning Circuit/1(I0 - VA)
  Outputs Signa Conditioning Circuit/8(Out 7) -> Mux1/8
  Outputs Signa Conditioning Circuit/6(Out 5) -> Mux1/6
  Constant3/1 -> Outputs Signa Conditioning Circuit/8(I7 - N/C)
  Constant1/1 -> Outputs Signa Conditioning Circuit/6(I5 - N/C)
  Outputs Signa Conditioning Circuit/1(Out 0) -> Mux1/1

== system IEEE_1547_UI_TEST/SM_SystemDynamics/PHIL SOFTWARE SIDE CURRENT SOURCES ==
  IA Cont. Sig : Inport
  IB Cont. Sig : Inport  Port=2
  IC Cont. Sig : Inport  Port=3
  Controlled Current Source3 : powerlib/Electrical Sources/Controlled Current Source  Initialize=off  Source_Type=AC  Amplitude=0  Phase=0  Frequency=0  Measurements=None
      settings: SourceProductName=Simscape Electrical
  Controlled Current Source4 : powerlib/Electrical Sources/Controlled Current Source  Initialize=off  Source_Type=AC  Amplitude=0  Phase=0  Frequency=0  Measurements=None
      settings: SourceProductName=Simscape Electrical
  Controlled Current Source5 : powerlib/Electrical Sources/Controlled Current Source  Initialize=off  Source_Type=AC  Amplitude=0  Phase=0  Frequency=0  Measurements=None
      settings: SourceProductName=Simscape Electrical
  Series RLC Branch1 : powerlib/Elements/Series RLC Branch  LConnTagsString=__new0  RConnTagsString=__new0  BranchType=R  Resistance=1e8  Inductance=1e-3  SetiL0=off  InitialCurrent=0  Capacitance=1e-6  Setx0=off  InitialVoltage=0  Measurements=None
      settings: SourceProductName=Simscape Electrical
  Series RLC Branch2 : powerlib/Elements/Series RLC Branch  LConnTagsString=__new0  RConnTagsString=__new0  BranchType=R  Resistance=1e8  Inductance=1e-3  SetiL0=off  InitialCurrent=0  Capacitance=1e-6  Setx0=off  InitialVoltage=0  Measurements=None
      settings: SourceProductName=Simscape Electrical
  Series RLC Branch3 : powerlib/Elements/Series RLC Branch  LConnTagsString=__new0  RConnTagsString=__new0  BranchType=R  Resistance=1e8  Inductance=1e-3  SetiL0=off  InitialCurrent=0  Capacitance=1e-6  Setx0=off  InitialVoltage=0  Measurements=None
      settings: SourceProductName=Simscape Electrical
  Subsystem : Subsystem
  Subsystem1 : Subsystem
  Subsystem2 : Subsystem
  Voltage Measurement3 : powerlib/Measurements/Voltage Measurement  PhasorSimulation=off  OutputType=Complex  PSBequivalent=0
      settings: SourceProductName=Simscape Electrical
  Voltage Measurement5 : powerlib/Measurements/Voltage Measurement  PhasorSimulation=off  OutputType=Complex  PSBequivalent=0
      settings: SourceProductName=Simscape Electrical
  Voltage Measurement6 : powerlib/Measurements/Voltage Measurement  PhasorSimulation=off  OutputType=Complex  PSBequivalent=0
      settings: SourceProductName=Simscape Electrical
  A : PMIOPort  Side=Left
  B : PMIOPort  Port=2  Side=Left
  C : PMIOPort  Tag=PMCPort  Port=3  Side=Left
  Gnd : PMIOPort  Port=4  Side=Left
  VA : Outport
  VB : Outport  Port=2
  VC : Outport  Port=3
  wires:
  Voltage Measurement6/1 -> VA/1
  Voltage Measurement5/1 -> VB/1
  Voltage Measurement3/1 -> VC/1
  IA Cont. Sig/1 -> Subsystem/2(input)
  IB Cont. Sig/1 -> Subsystem1/2(input)
  IC Cont. Sig/1 -> Subsystem2/2(input)
  [stop_ametek] -> Subsystem/1(trig)
  Subsystem/1(Out1) -> Controlled Current Source5/1
  [stop_ametek] -> Subsystem1/1(trig)
  Subsystem1/1(Out1) -> Controlled Current Source4/1
  [stop_ametek] -> Subsystem2/1(trig)
  Subsystem2/1(Out1) -> Controlled Current Source3/1
  connections:
  Controlled Current Source3/RConn1 -- Series RLC Branch1/RConn1 -- C/RConn1 -- Voltage Measurement3/LConn1
  Controlled Current Source5/LConn1 -- Voltage Measurement6/LConn2 -- Series RLC Branch3/LConn1 -- Controlled Current Source4/LConn1 -- Series RLC Branch2/LConn1 -- Voltage Measurement3/LConn2 -- Controlled Current Source3/LConn1 -- Series RLC Branch1/LConn1 -- Gnd/RConn1 -- Voltage Measurement5/LConn2
  Series RLC Branch2/RConn1 -- Controlled Current Source4/RConn1 -- Voltage Measurement5/LConn1 -- B/RConn1
  Series RLC Branch3/RConn1 -- Controlled Current Source5/RConn1 -- Voltage Measurement6/LConn1 -- A/RConn1

== system IEEE_1547_UI_TEST/SM_SystemDynamics/RLC values ==
  note: RESISTOR
  note: INDUCTOR
  note: CAPACITOR
  Subsystem : Subsystem
      mask Display: color('black');disp('Resistor\nBank\nAdjust')
  Subsystem1 : Subsystem
      mask Display: color('black'), disp('Rinternal\nBank\nAdjust')
  Subsystem2 : Subsystem
      mask Display: color('black'),disp('Inductor\nBank\nAdjust')
  Subsystem3 : Subsystem
      mask Display: color('black'),disp('Capacitor\nBank\nAdjust')

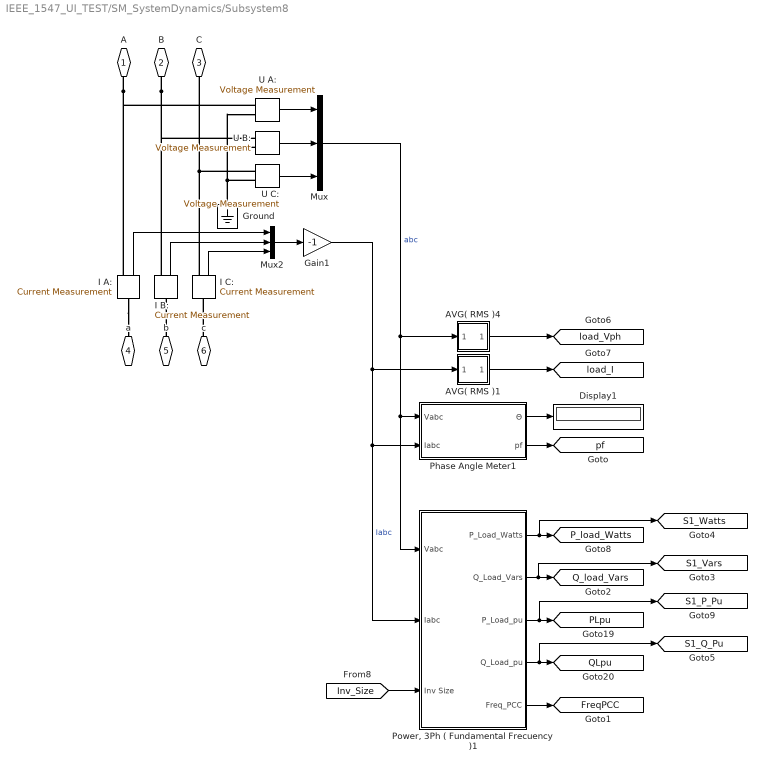
== system IEEE_1547_UI_TEST/SM_SystemDynamics/Subsystem8 ==
  AVG( RMS )1 : Subsystem
      mask Display: color('blue');disp('RMS\nAVG')
  AVG( RMS )4 : Subsystem
      mask Display: color('blue');disp('RMS\nAVG')
  Display1 : Display
  Gain1 : Gain  Gain=-1
  Ground : powerlib/Elements/Ground  LConnTagsString=a
  I A: : powerlib/Measurements/Current Measurement  PhasorSimulation=off  OutputType=Complex  PSBequivalent=0
  I B: : powerlib/Measurements/Current Measurement  PhasorSimulation=off  OutputType=Complex  PSBequivalent=0
  I C: : powerlib/Measurements/Current Measurement  PhasorSimulation=off  OutputType=Complex  PSBequivalent=0
  Mux : Mux  Inputs=3
  Mux2 : Mux  Inputs=3
  Phase Angle Meter1 : Subsystem
      mask Display:
      | color('blue')
      | disp('Θ = (Θv - Θi)')
  "Power, 3Ph ( Fundamental Frecuency )1" : Subsystem
  U A: : powerlib/Measurements/Voltage Measurement  PhasorSimulation=off  OutputType=Complex  PSBequivalent=0
  U B: : powerlib/Measurements/Voltage Measurement  PhasorSimulation=off  OutputType=Complex  PSBequivalent=0
  U C: : powerlib/Measurements/Voltage Measurement  PhasorSimulation=off  OutputType=Complex  PSBequivalent=0
  A : PMIOPort  Side=Left
  B : PMIOPort  Port=2  Side=Left
  C : PMIOPort  Port=3  Side=Left
  a : PMIOPort  Port=4  Side=Right
  b : PMIOPort  Port=5  Side=Right
  c : PMIOPort  Port=6  Side=Right
  tag scope: FreqPCC=global, PLpu=global, P_load_Watts=global, QLpu=global, Q_load_Vars=global, S1_P_Pu=global, S1_Q_Pu=global, S1_Vars=global, S1_Watts=global, load_I=global, load_Vph=global, pf=global
  wires:
  I B:/1 -> Mux2/2
  I C:/1 -> Mux2/3
  U A:/1 -> Mux/1
  U B:/1 -> Mux/2
  I A:/1 -> Mux2/1
  U C:/1 -> Mux/3
  Mux2/1 -> Gain1/1
  Phase Angle Meter1/2(pf) -> [pf]
  Mux/1 -> "Power, 3Ph ( Fundamental Frecuency )1"/1(Vabc), Phase Angle Meter1/1(Vabc), AVG( RMS )4/1(In1)  "abc"
  Gain1/1 -> AVG( RMS )1/1(In1), "Power, 3Ph ( Fundamental Frecuency )1"/2(Iabc), Phase Angle Meter1/2(Iabc)  "Iabc"
  [Inv_Size] -> "Power, 3Ph ( Fundamental Frecuency )1"/3(Inv Size)
  Phase Angle Meter1/1(Θ) -> Display1/1
  AVG( RMS )4/1(Out1) -> [load_Vph]
  AVG( RMS )1/1(Out1) -> [load_I]
  "Power, 3Ph ( Fundamental Frecuency )1"/4(Q_Load_pu) -> [S1_Q_Pu], [QLpu]
  "Power, 3Ph ( Fundamental Frecuency )1"/1(P_Load_Watts) -> [S1_Watts], [P_load_Watts]
  "Power, 3Ph ( Fundamental Frecuency )1"/3(P_Load_pu) -> [S1_P_Pu], [PLpu]
  "Power, 3Ph ( Fundamental Frecuency )1"/5(Freq_PCC) -> [FreqPCC]
  "Power, 3Ph ( Fundamental Frecuency )1"/2(Q_Load_Vars) -> [S1_Vars], [Q_load_Vars]
  connections:
  B/RConn1 -- I B:/RConn1 -- U B:/LConn1
  U C:/LConn2 -- U A:/LConn2 -- U B:/LConn2 -- Ground/LConn1
  A/RConn1 -- I A:/RConn1 -- U A:/LConn1
  I C:/RConn1 -- U C:/LConn1 -- C/RConn1
  b/RConn1 -- I B:/LConn1
  c/RConn1 -- I C:/LConn1
  I A:/LConn1 -- a/RConn1

== system IEEE_1547_UI_TEST/SM_SystemDynamics/UTILITY1 ==
  AVG( RMS )4 : Subsystem
      mask Display: color('blue');disp('RMS\nAVG')
  AVG( RMS )5 : Subsystem
      mask Display: color('blue');disp('RMS\nAVG')
  "Power, 3Ph ( Fundamental Frecuency )2" : Subsystem
  Three-Phase V-I Measurement From EPS : powerlib/Measurements/Three-Phase V-I Measurement  VoltageMeasurement=phase-to-ground  SetLabelV=off  LabelV=Vabc_INV  Vpu=off  VpuLL=off  CurrentMeasurement=yes  SetLabelI=off  LabelI=Iabc_INV  Ipu=off  Pbase=100e6  Vbase=500e3  OutputType=Complex  PhasorSimulation=off  PSBequivalent=0
      settings: SourceProductName=Simscape Electrical
  A : PMIOPort  Side=Left
  B : PMIOPort  Port=2  Side=Left
  C : PMIOPort  Port=3  Side=Left
  a : PMIOPort  Port=4  Side=Right
  b : PMIOPort  Port=5  Side=Right
  c : PMIOPort  Port=6  Side=Right
  tag scope: Freq_EPS=global, Puti_Watts=global, Puti_pu=global, Quti_Vars=global, Quti_pu=global, S3_P_Pu=global, S3_Q_Pu=global, S3_Vars=global, S3_Watts=global, Vph_Uti=global, uti_I=global
  wires:
  AVG( RMS )4/1(Out1) -> [Vph_Uti]
  AVG( RMS )5/1(Out1) -> [uti_I]
  [Inv_Size] -> "Power, 3Ph ( Fundamental Frecuency )2"/3(Inv Size)
  Three-Phase V-I Measurement From EPS/2 -> "Power, 3Ph ( Fundamental Frecuency )2"/2(Iabc), AVG( RMS )5/1(In1)  "Iabc"
  Three-Phase V-I Measurement From EPS/1 -> "Power, 3Ph ( Fundamental Frecuency )2"/1(Vabc), AVG( RMS )4/1(In1)  "Vabc"
  "Power, 3Ph ( Fundamental Frecuency )2"/4(Quti_pu) -> [S3_Q_Pu], [Quti_pu]
  "Power, 3Ph ( Fundamental Frecuency )2"/5(Freq_EPS) -> [Freq_EPS]
  "Power, 3Ph ( Fundamental Frecuency )2"/3(Puti_pu) -> [S3_P_Pu], [Puti_pu]
  "Power, 3Ph ( Fundamental Frecuency )2"/2(Quti_Vars) -> [S3_Vars], [Quti_Vars]
  "Power, 3Ph ( Fundamental Frecuency )2"/1(Pt_uti_Watts) -> [S3_Watts], [Puti_Watts]
  connections:
  Three-Phase V-I Measurement From EPS/RConn3 -- c/RConn1
  C/RConn1 -- Three-Phase V-I Measurement From EPS/LConn3
  Three-Phase V-I Measurement From EPS/RConn2 -- b/RConn1
  B/RConn1 -- Three-Phase V-I Measurement From EPS/LConn2
  A/RConn1 -- Three-Phase V-I Measurement From EPS/LConn1
  Three-Phase V-I Measurement From EPS/RConn1 -- a/RConn1

== system IEEE_1547_UI_TEST/SC_InputsandOutputs/Subsystem9/Subsystem5 ==
  Utility Measurements : Inport
  Bus Selector : BusSelector  OutputSignals=Utility VLL,Utility I,Utility Ppu,Utility Qpu
  To Workspace : ToWorkspace  VariableName=Uti_VLL  SaveFormat=Timeseries  SampleTime=-1
  To Workspace1 : ToWorkspace  VariableName=Uti_I  SaveFormat=Timeseries  SampleTime=-1
  To Workspace2 : ToWorkspace  VariableName=Uti_Ptot_pu  SaveFormat=Timeseries  SampleTime=-1
  To Workspace3 : ToWorkspace  VariableName=Uti_Qtot_pu  SaveFormat=Timeseries  SampleTime=-1
  wires:
  Utility Measurements/1 -> Bus Selector/1
  Bus Selector/1 -> To Workspace/1  "<Utility VLL>"
  Bus Selector/2 -> To Workspace1/1  "<Utility I>"
  Bus Selector/3 -> To Workspace2/1  "<Utility Ppu>"
  Bus Selector/4 -> To Workspace3/1  "<Utility Qpu>"
